simulink model "RoboSoccer"  (R2021b)
settings: Solver=ode15s  StartTime=0.0  StopTime=inf  RelTol=1e-3  EnableMultiTasking=on
PreLoadFcn:
  | load busobjects.mat;
libraries: vrlib x6, simulink x4
settings Model: Creator=smahapat  LastModifiedBy=sarth
settings SolverCC: ZeroCrossControl=DisableAll  AlgebraicLoopSolver=TrustRegion
settings DataIOCC: LimitDataPoints=on  SaveFormat=Array  SignalLoggingSaveFormat=ModelDataLogs  ReturnWorkspaceOutputs=off
settings OptimizationCC: DefaultParameterBehavior=Inlined  ExpressionDepthLimit=2147483647  LifeSpan=inf
settings DebuggingCC: UnderspecifiedInitializationDetection=Classic  MergeDetectMultiDrivingBlocksExec=none  SolverPrmCheckMsg=warning  FcnCallInpInsideContextMsg=warning  StateNameClashWarn=warning  SFUnexpectedBacktrackingDiag=warning  SFNoUnconditionalDefaultTransitionDiag=warning  SFExecutionAtInitializationDiag=none  SFMachineParentedDataDiag=warning  ArithmeticOperatorsInVariantConditions=warning
settings HardwareCC: ProdBitPerPointer=32  ProdBitPerSizeT=32  ProdBitPerPtrDiffT=32  ProdLargestAtomicFloat=None  ProdIntDivRoundTo=Undefined  ProdEndianess=Unspecified  ProdWordSize=32  ProdHWDeviceType=32-bit Generic
settings ModelReferenceCC: PropagateSignalLabelsOutOfModel=off
settings SFSimCC: SimUseLocalCustomCode=off  SimParseCustomCode=off  CustomCodeUndefinedFunction=UseInterfaceOnly
settings RTWCC: RTWUseLocalCustomCode=off
settings CodeAppCC: StateflowObjectComments=on
settings GRTTargetCC: TargetLangStandard=C89/C90 (ANSI)  CombineOutputUpdateFcns=off  GRTInterface=on
settings ConfigComp: CovMetricSettings=dw  CovSaveCumulativeToWorkspaceVar=on  CovSaveSingleToWorkspaceVar=on  CovExternalEMLEnable=off

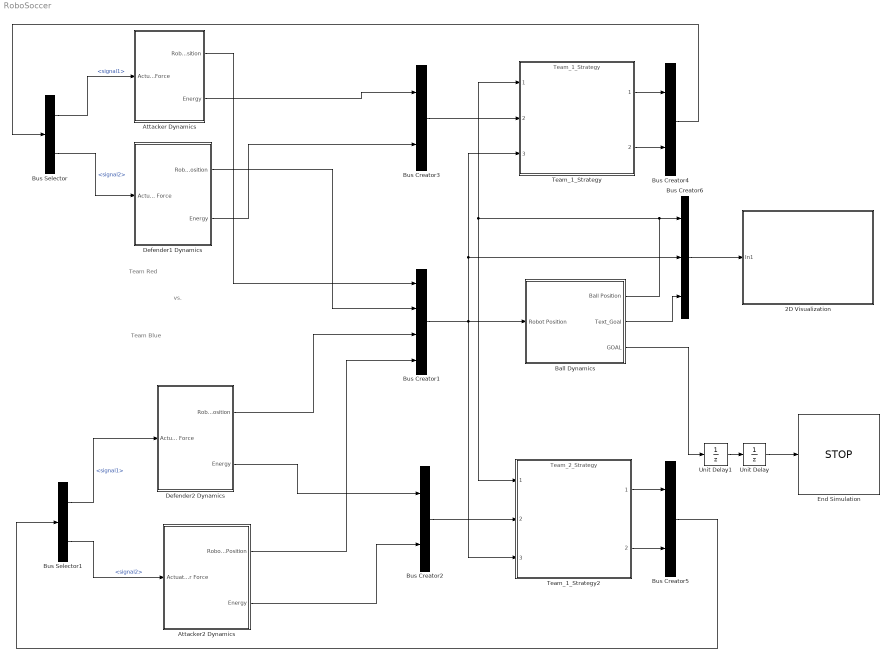
== system RoboSoccer ==
  note: Team Blue
  note: Team Red
  note: vs.
  2D Visualization : Subsystem
      mask Display: image(imread('texture\3D_visualization.jpg'));
  Attacker Dynamics : Subsystem  mask(Robot Parameters){P=0.5, saturate_value=0}
      mask prompts: P "Stamina (Enter value between 0 and 1)"; saturate_value "Actuator_saturation"
      mask help:
      | Set the robot stamina to a value between 0.1 and 1. Note that a higher value of stamina corresponds to more battery power which inversely impacts the mass of the robot. This will reduce its agility.
      |
      | Likewise, higher values of accuracy will come at a cost of higher rates of discharge for the battery pack.
      |
      | Choose values carefully to reflect these tradeoffs.
      mask init:
      | saturate_value=300;
      settings: CloseFcn=|
      | if P<0
      |     error('P cannot be less than 0');
      | end
      | if P>1
      |     error('P cannot be greater than 1');
      | end
      | 
      | if sigma<0
      |     error('sigma cannot be less than 0');
      | end
      | 
      | if sigma>1
      |     error('sigma cannot be greater than 1');
      | end
      mask Help:
      | Set the robot stamina to a value between 0.1 and 1. Note that a higher value of stamina corresponds to more battery power which inversely impacts the mass of the robot. This will reduce its agility.
      | 
      | Likewise, higher values of accuracy will come at a cost of higher rates of discharge for the battery pack.
      | 
      | Choose values carefully to reflect these tradeoffs.
      mask Callback saturate_value: saturate_value=10;
      mask Display: image(imread('texture\Nao6_D.jpeg'));
  Attacker2 Dynamics : Subsystem  mask(Robot Parameters){P=0.5, saturate_value=0}
      mask prompts: P "Stamina (Enter value between 0 and 1)"; saturate_value "Actuator_saturation"
      mask help:
      | Set the robot stamina to a value between 0.1 and 1. Note that a higher value of stamina corresponds to more battery power which inversely impacts the mass of the robot. This will reduce its agility.
      |
      | Likewise, higher values of accuracy will come at a cost of higher rates of discharge for the battery pack.
      |
      | Choose values carefully to reflect these tradeoffs.
      mask init:
      | saturate_value=300;
      settings: CloseFcn=|
      | if P<0
      |     error('P cannot be less than 0');
      | end
      | if P>1
      |     error('P cannot be greater than 1');
      | end
      | 
      | if sigma<0
      |     error('sigma cannot be less than 0');
      | end
      | 
      | if sigma>1
      |     error('sigma cannot be greater than 1');
      | end
      mask Help:
      | Set the robot stamina to a value between 0.1 and 1. Note that a higher value of stamina corresponds to more battery power which inversely impacts the mass of the robot. This will reduce its agility.
      | 
      | Likewise, higher values of accuracy will come at a cost of higher rates of discharge for the battery pack.
      | 
      | Choose values carefully to reflect these tradeoffs.
      mask Callback saturate_value: saturate_value=10;
      mask Display: image(imread('texture\Nao6_D.jpeg'));
  Ball Dynamics : Subsystem  TreatAsAtomicUnit=on
      mask Display: image(imread('texture\soccer_ball_dynamics.jpg'));
  Bus Creator1 : BusCreator  Inputs=4  OutDataTypeStr=Bus: Bus_Robot_Positions
  Bus Creator2 : BusCreator  Inputs=2  OutDataTypeStr=Bus: Bus_Power
  Bus Creator3 : BusCreator  Inputs=2  OutDataTypeStr=Bus: Bus_Power
  Bus Creator4 : BusCreator  Inputs=2
  Bus Creator5 : BusCreator  Inputs=2
  Bus Creator6 : BusCreator  Inputs=3
  Bus Selector : BusSelector  OutputSignals=signal1,signal2
  Bus Selector1 : BusSelector  OutputSignals=signal1,signal2
  Defender1 Dynamics : Subsystem  mask(Robot Parameters){P=0.5, saturate_value=0}
      mask prompts: P "Stamina (Enter value between 0 and 1)"; saturate_value "Actuator_saturation"
      mask help:
      | Set the robot stamina to a value between 0.1 and 1. Note that a higher value of stamina corresponds to more battery power which inversely impacts the mass of the robot. This will reduce its agility.
      |
      | Likewise, higher values of accuracy will come at a cost of higher rates of discharge for the battery pack.
      |
      | Choose values carefully to reflect these tradeoffs.
      mask init:
      | saturate_value=300;
      settings: CloseFcn=|
      | if P<0
      |     error('P cannot be less than 0');
      | end
      | if P>1
      |     error('P cannot be greater than 1');
      | end
      | 
      | if sigma<0
      |     error('sigma cannot be less than 0');
      | end
      | 
      | if sigma>1
      |     error('sigma cannot be greater than 1');
      | end
      mask Help:
      | Set the robot stamina to a value between 0.1 and 1. Note that a higher value of stamina corresponds to more battery power which inversely impacts the mass of the robot. This will reduce its agility.
      | 
      | Likewise, higher values of accuracy will come at a cost of higher rates of discharge for the battery pack.
      | 
      | Choose values carefully to reflect these tradeoffs.
      mask Callback saturate_value: saturate_value=10;
      mask Display: image(imread('texture\Nao6_A.jpeg'));
  Defender2 Dynamics : Subsystem  mask(Robot Parameters){P=0.5, saturate_value=0}
      mask prompts: P "Stamina (Enter value between 0 and 1)"; saturate_value "Actuator_saturation"
      mask help:
      | Set the robot stamina to a value between 0.1 and 1. Note that a higher value of stamina corresponds to more battery power which inversely impacts the mass of the robot. This will reduce its agility.
      |
      | Likewise, higher values of accuracy will come at a cost of higher rates of discharge for the battery pack.
      |
      | Choose values carefully to reflect these tradeoffs.
      mask init:
      | saturate_value=300;
      settings: CloseFcn=|
      | if P<0
      |     error('P cannot be less than 0');
      | end
      | if P>1
      |     error('P cannot be greater than 1');
      | end
      | 
      | if sigma<0
      |     error('sigma cannot be less than 0');
      | end
      | 
      | if sigma>1
      |     error('sigma cannot be greater than 1');
      | end
      mask Help:
      | Set the robot stamina to a value between 0.1 and 1. Note that a higher value of stamina corresponds to more battery power which inversely impacts the mass of the robot. This will reduce its agility.
      | 
      | Likewise, higher values of accuracy will come at a cost of higher rates of discharge for the battery pack.
      | 
      | Choose values carefully to reflect these tradeoffs.
      mask Callback saturate_value: saturate_value=10;
      mask Display: image(imread('texture\Nao6_A.jpeg'));
  End Simulation : Stop
  Team_1_Strategy : ModelReference  ModelNameDialog=Team_1_Strategy  SimulationMode=Normal  ModelReferenceVersion=1.19
      mask Display: image(imread('texture\Strategy.jpg'));
  Team_1_Strategy2 : ModelReference  ModelNameDialog=Team_2_Strategy  SimulationMode=Normal  ModelReferenceVersion=1.24
      mask Display: image(imread('texture\strategy.jpg'));
  Unit Delay : UnitDelay  SampleTime=-1
  Unit Delay1 : UnitDelay  SampleTime=-1
  wires:
  Attacker Dynamics/1(Robot Position) -> Bus Creator1/1
  Defender1 Dynamics/1(Robot Position) -> Bus Creator1/2
  Defender2 Dynamics/1(Robot Position) -> Bus Creator1/3
  Attacker2 Dynamics/1(Robot Position) -> Bus Creator1/4
  Bus Creator1/1 -> Ball Dynamics/1(Robot Position), Bus Creator6/2, Team_1_Strategy/3, Team_1_Strategy2/3
  Defender2 Dynamics/2(Energy) -> Bus Creator2/1
  Attacker2 Dynamics/2(Energy) -> Bus Creator2/2
  Bus Creator2/1 -> Team_1_Strategy2/2
  Team_1_Strategy2/1 -> Bus Creator5/1
  Team_1_Strategy2/2 -> Bus Creator5/2
  Bus Creator5/1 -> Bus Selector1/1
  Team_1_Strategy/1 -> Bus Creator4/1
  Team_1_Strategy/2 -> Bus Creator4/2
  Bus Creator4/1 -> Bus Selector/1
  Bus Selector/1 -> Attacker Dynamics/1(Actuator Force)  "<signal1>"
  Bus Selector/2 -> Defender1 Dynamics/1(Actuator Force)  "<signal2>"
  Bus Selector1/1 -> Defender2 Dynamics/1(Actuator Force)  "<signal1>"
  Bus Selector1/2 -> Attacker2 Dynamics/1(Actuator Force)  "<signal2>"
  Ball Dynamics/3(GOAL) -> Unit Delay1/1
  Ball Dynamics/1(Ball Position) -> Bus Creator6/1, Team_1_Strategy/1, Team_1_Strategy2/1
  Bus Creator6/1 -> 2D Visualization/1(In1)
  Ball Dynamics/2(Text_Goal) -> Bus Creator6/3
  Bus Creator3/1 -> Team_1_Strategy/2
  Defender1 Dynamics/2(Energy) -> Bus Creator3/2
  Attacker Dynamics/2(Energy) -> Bus Creator3/1
  Unit Delay/1 -> End Simulation/1
  Unit Delay1/1 -> Unit Delay/1

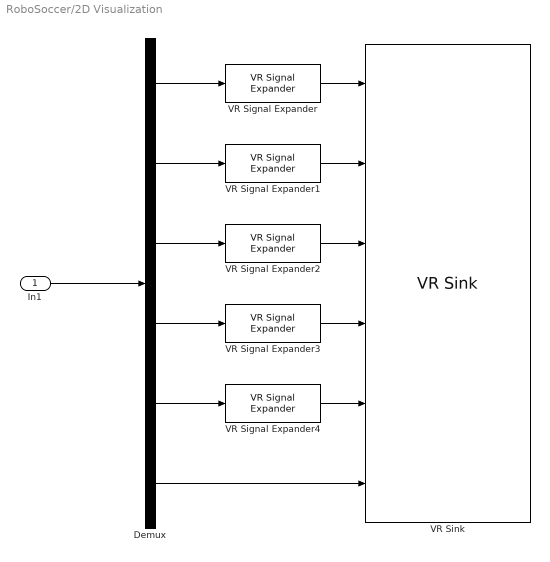
== system RoboSoccer/2D Visualization ==
  In1 : Inport
  Demux : Demux  Outputs=6
  VR Signal Expander{,1..4} (5 alike) : vrlib/VR Signal Expander  outwidth=3  outidx=[1 2]
  VR Sink : vrlib/VR Sink  InstantiateOnLoad=on  SampleTime=0.01  ViewEnable=on  RemoteChange=off  RemoteView=on  FieldsWritten=Ball.translation.3.1.1.double#Robot_1.translation.3.1.1.double#Robot_2.translation.3.1.1.double#Robot_3.translation.3.1.1.double#Robot_4.translation.3.1.1.double#GOAL.translation.3.1.1.double  WorldFileName=robosoccer.WRL  WorldDescription=Robot Soccer Simulator  AutoView=on  VideoDimensions=[]  AllowVariableSize=off
  wires:
  VR Signal Expander/1 -> VR Sink/1
  VR Signal Expander1/1 -> VR Sink/2
  VR Signal Expander2/1 -> VR Sink/3
  VR Signal Expander4/1 -> VR Sink/5
  In1/1 -> Demux/1
  Demux/5 -> VR Signal Expander4/1
  Demux/4 -> VR Signal Expander3/1
  Demux/3 -> VR Signal Expander2/1
  Demux/2 -> VR Signal Expander1/1
  Demux/1 -> VR Signal Expander/1
  VR Signal Expander3/1 -> VR Sink/4
  Demux/6 -> VR Sink/6

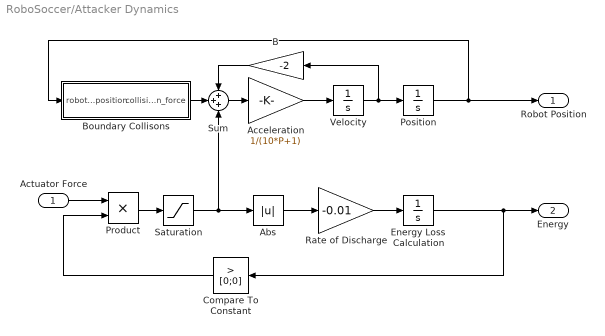
== system RoboSoccer/Attacker Dynamics ==
  Actuator Force : Inport
  Abs : Abs
  Acceleration : Gain  Gain=1/(10*P+1)
  B : Gain  Gain=-2
  Boundary Collisons : MATLAB Function  TreatAsAtomicUnit=on
  Compare To Constant : simulink/Logic and Bit Operations/Compare To Constant  relop=>  const=[0;0]  OutDataTypeStr=uint8
  Energy Loss Calculation : Integrator  InitialCondition=1000*[P; P]
  Position : Integrator  InitialCondition=[50; 75]
  Product : Product  RndMeth=Zero
  Rate of Discharge : Gain  Gain=-0.01
  Saturation : Saturate  UpperLimit=saturate_value  LowerLimit=-saturate_value
  Sum : Sum  Inputs=+++
  Velocity : Integrator  InitialCondition=[0;0]
  Robot Position : Outport  PortDimensions=[2 1]
  Energy : Outport  Port=2  PortDimensions=[2 1]
  wires:
  Acceleration/1 -> Velocity/1
  Velocity/1 -> Position/1, B/1
  Position/1 -> Boundary Collisons/1(robot_position), Robot Position/1
  Energy Loss Calculation/1 -> Energy/1, Compare To Constant/1
  Rate of Discharge/1 -> Energy Loss Calculation/1
  Saturation/1 -> Abs/1, Sum/3
  Abs/1 -> Rate of Discharge/1
  Actuator Force/1 -> Product/1
  Product/1 -> Saturation/1
  Compare To Constant/1 -> Product/2
  Boundary Collisons/1(collision_force) -> Sum/2
  Sum/1 -> Acceleration/1
  B/1 -> Sum/1

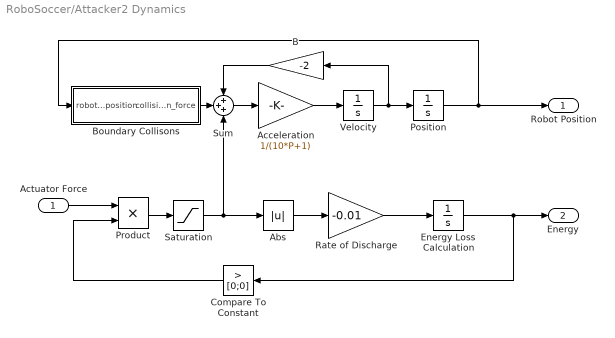
== system RoboSoccer/Attacker2 Dynamics ==
  Actuator Force : Inport
  Abs : Abs
  Acceleration : Gain  Gain=1/(10*P+1)
  B : Gain  Gain=-2
  Boundary Collisons : MATLAB Function  TreatAsAtomicUnit=on
  Compare To Constant : simulink/Logic and Bit Operations/Compare To Constant  relop=>  const=[0;0]  OutDataTypeStr=uint8
  Energy Loss Calculation : Integrator  InitialCondition=1000*[P; P]
  Position : Integrator  InitialCondition=[150; 25]
  Product : Product  RndMeth=Zero
  Rate of Discharge : Gain  Gain=-0.01
  Saturation : Saturate  UpperLimit=saturate_value  LowerLimit=-saturate_value
  Sum : Sum  Inputs=+++
  Velocity : Integrator  InitialCondition=[0;0]
  Robot Position : Outport  PortDimensions=[2 1]
  Energy : Outport  Port=2  PortDimensions=[2 1]
  wires:
  Sum/1 -> Acceleration/1
  Acceleration/1 -> Velocity/1
  Velocity/1 -> Position/1, B/1
  Position/1 -> Boundary Collisons/1(robot_position), Robot Position/1
  Energy Loss Calculation/1 -> Energy/1, Compare To Constant/1
  Rate of Discharge/1 -> Energy Loss Calculation/1
  Saturation/1 -> Abs/1, Sum/3
  Abs/1 -> Rate of Discharge/1
  Actuator Force/1 -> Product/1
  Product/1 -> Saturation/1
  Compare To Constant/1 -> Product/2
  Boundary Collisons/1(collision_force) -> Sum/2
  B/1 -> Sum/1

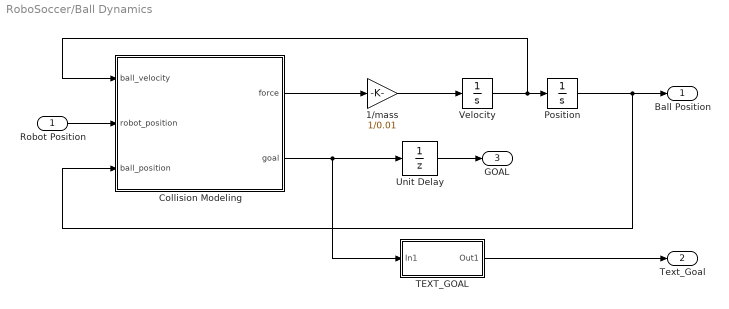
== system RoboSoccer/Ball Dynamics ==
  Robot Position : Inport
  1/mass : Gain  Gain=1/0.01
  Collision Modeling : MATLAB Function  TreatAsAtomicUnit=on
  Position : Integrator  InitialCondition=[100;50]
  TEXT_GOAL : Subsystem
  Unit Delay : UnitDelay  SampleTime=-1
  Velocity : Integrator  InitialCondition=[0;0]
  Ball Position : Outport
  Text_Goal : Outport  Port=2
  GOAL : Outport  Port=3
  wires:
  Robot Position/1 -> Collision Modeling/2(robot_position)
  Velocity/1 -> Position/1, Collision Modeling/1(ball_velocity)
  Position/1 -> Ball Position/1, Collision Modeling/3(ball_position)
  Collision Modeling/1(force) -> 1/mass/1
  1/mass/1 -> Velocity/1
  Collision Modeling/2(goal) -> Unit Delay/1, TEXT_GOAL/1(In1)
  Unit Delay/1 -> GOAL/1
  TEXT_GOAL/1(Out1) -> Text_Goal/1

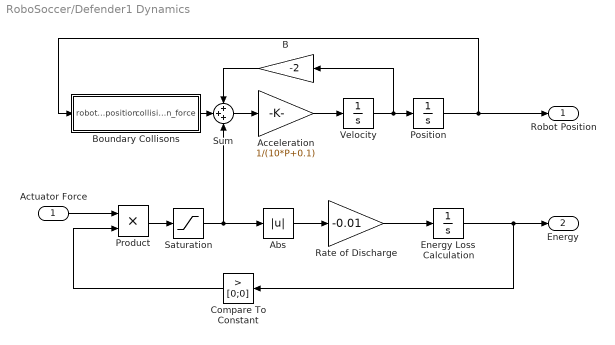
== system RoboSoccer/Defender1 Dynamics ==
  Actuator Force : Inport
  Abs : Abs
  Acceleration : Gain  Gain=1/(10*P+0.1)
  B : Gain  Gain=-2
  Boundary Collisons : MATLAB Function  TreatAsAtomicUnit=on
  Compare To Constant : simulink/Logic and Bit Operations/Compare To Constant  relop=>  const=[0;0]  OutDataTypeStr=uint8
  Energy Loss Calculation : Integrator  InitialCondition=1000*[P; P]
  Position : Integrator  InitialCondition=[50; 25]
  Product : Product  RndMeth=Zero
  Rate of Discharge : Gain  Gain=-0.01
  Saturation : Saturate  UpperLimit=saturate_value  LowerLimit=-saturate_value
  Sum : Sum  Inputs=+++
  Velocity : Integrator  InitialCondition=[0;0]
  Robot Position : Outport  PortDimensions=[2 1]
  Energy : Outport  Port=2  PortDimensions=[2 1]
  wires:
  Compare To Constant/1 -> Product/2
  Product/1 -> Saturation/1
  Actuator Force/1 -> Product/1
  Abs/1 -> Rate of Discharge/1
  Saturation/1 -> Abs/1, Sum/3
  Rate of Discharge/1 -> Energy Loss Calculation/1
  Energy Loss Calculation/1 -> Compare To Constant/1, Energy/1
  Position/1 -> Robot Position/1, Boundary Collisons/1(robot_position)
  Velocity/1 -> Position/1, B/1
  Acceleration/1 -> Velocity/1
  Sum/1 -> Acceleration/1
  Boundary Collisons/1(collision_force) -> Sum/2
  B/1 -> Sum/1

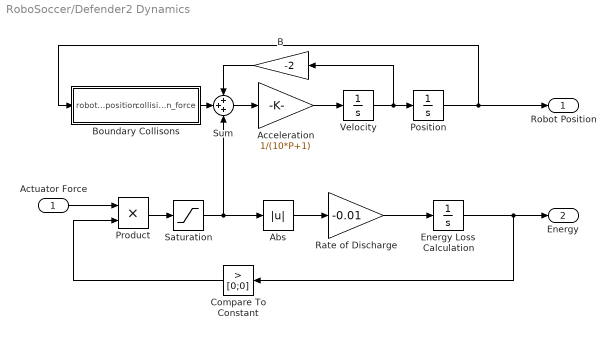
== system RoboSoccer/Defender2 Dynamics ==
  Actuator Force : Inport
  Abs : Abs
  Acceleration : Gain  Gain=1/(10*P+1)
  B : Gain  Gain=-2
  Boundary Collisons : MATLAB Function  TreatAsAtomicUnit=on
  Compare To Constant : simulink/Logic and Bit Operations/Compare To Constant  relop=>  const=[0;0]  OutDataTypeStr=uint8
  Energy Loss Calculation : Integrator  InitialCondition=1000*[P; P]
  Position : Integrator  InitialCondition=[150; 75]
  Product : Product  RndMeth=Zero
  Rate of Discharge : Gain  Gain=-0.01
  Saturation : Saturate  UpperLimit=saturate_value  LowerLimit=-saturate_value
  Sum : Sum  Inputs=+++
  Velocity : Integrator  InitialCondition=[0;0]
  Robot Position : Outport  PortDimensions=[2 1]
  Energy : Outport  Port=2  PortDimensions=[2 1]
  wires:
  Compare To Constant/1 -> Product/2
  Product/1 -> Saturation/1
  Actuator Force/1 -> Product/1
  Abs/1 -> Rate of Discharge/1
  Saturation/1 -> Abs/1, Sum/3
  Rate of Discharge/1 -> Energy Loss Calculation/1
  Energy Loss Calculation/1 -> Compare To Constant/1, Energy/1
  Position/1 -> Robot Position/1, Boundary Collisons/1(robot_position)
  Velocity/1 -> Position/1, B/1
  Acceleration/1 -> Velocity/1
  Sum/1 -> Acceleration/1
  Boundary Collisons/1(collision_force) -> Sum/2
  B/1 -> Sum/1

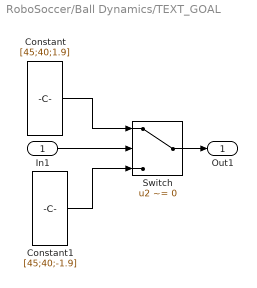
== system RoboSoccer/Ball Dynamics/TEXT_GOAL ==
  In1 : Inport
  Constant : Constant  Value=[45;40;1.9]
  Constant1 : Constant  Value=[45;40;-1.9]
  Switch : Switch  Criteria=u2 ~= 0  Threshold=1
  Out1 : Outport
  wires:
  In1/1 -> Switch/2
  Switch/1 -> Out1/1
  Constant/1 -> Switch/1
  Constant1/1 -> Switch/3

== matlab function RoboSoccer/Ball Dynamics/Collision Modeling ==
  data: ball_velocity input; robot_position input size=[8 ;1]; ball_position input size=[2;1]; force output size=[2;1]; goal output
function [force, goal] = fcn(ball_velocity,robot_position, ball_position)
%#eml
% Initialize variables

force1=zeros(2,1);
force2=zeros(2,1);
force3=zeros(2,1);
force4=zeros(2,1);
collision_force=zeros(2,1);
d1=zeros(2,1);
d2=zeros(2,1);
d3=zeros(2,1);
d4=zeros(2,1);
K=100;
goal=0;
tol=25;
B=0.01;

% Compute dot products and calculate impulsive forces on the ball
d1=robot_position(1:2,1)-ball_position;
d2=robot_position(3:4,1)-ball_position;
d3=robot_position(5:6,1)-ball_position;
d4=robot_position(7:8,1)-ball_position;

if   dot(d1,d1) <tol
     force1=-K*d1;
end

if   dot(d2,d2) <tol
     force2=-K*d2;
end

if   dot(d3,d3) <tol
     force3=-K*d3;
end

if   dot(d4,d4) <tol
     force4=-K*d4;
end

% Code to check for boundary collisions for the ball
if ball_position(1,1)<0 
    collision_force(1,1)=-K*ball_position(1,1);
end

if ball_position(1,1)>200 
    collision_force(1,1)=K*(200-ball_position(1,1));
end

if ball_position(2,1)<0 
    collision_force(2,1)=-K*ball_position(2,1);
end

if ball_position(2,1)>100 
    collision_force(2,1)=K*(100-ball_position(2,1)); 
end

% Total force
force=collision_force+force1+force2+force3+force4-B*ball_velocity;

% Goal scored
if ((ball_position(1,1)<=0) && (ball_position(2,1)>41) && (ball_position(2,1)<59))
    goal=1; 
end

if ((ball_position(1,1)>=200) && (ball_position(2,1)>41) && (ball_position(2,1)<59))
    goal=1; 
end

== matlab function RoboSoccer/Attacker Dynamics/Boundary Collisons ==
  data: robot_position input; collision_force output
function collision_force = fcn(robot_position)
%#eml
K=100;
collision_force=[0; 0]; 
if robot_position(1,1)<0 
    collision_force(1,1)=-K*robot_position(1,1);
end

if robot_position(1,1)>200 
    collision_force(1,1)=K*(200-robot_position(1,1));
end

if robot_position(2,1)<0 
    collision_force(2,1)=-K*robot_position(2,1);
end

if robot_position(2,1)>100 
    collision_force(2,1)=K*(100-robot_position(2,1));
end

== matlab function RoboSoccer/Attacker2 Dynamics/Boundary Collisons ==
  data: robot_position input; collision_force output
function collision_force = fcn(robot_position)
%#eml
K=100;
collision_force=[0; 0]; 
if robot_position(1,1)<0 
    collision_force(1,1)=-K*robot_position(1,1);
end

if robot_position(1,1)>200 
    collision_force(1,1)=K*(200-robot_position(1,1));
end

if robot_position(2,1)<0 
    collision_force(2,1)=-K*robot_position(2,1);
end

if robot_position(2,1)>100 
    collision_force(2,1)=K*(100-robot_position(2,1));
end

== matlab function RoboSoccer/Defender2 Dynamics/Boundary Collisons ==
  data: robot_position input; collision_force output
function collision_force = fcn(robot_position)
%#eml
K=100;
collision_force=[0; 0]; 
if robot_position(1,1)<0 
    collision_force(1,1)=-K*robot_position(1,1);
end

if robot_position(1,1)>200 
    collision_force(1,1)=K*(200-robot_position(1,1));
end

if robot_position(2,1)<0 
    collision_force(2,1)=-K*robot_position(2,1);
end

if robot_position(2,1)>100 
    collision_force(2,1)=K*(100-robot_position(2,1));
end

== matlab function RoboSoccer/Defender1 Dynamics/Boundary Collisons ==
  data: robot_position input; collision_force output
function collision_force = fcn(robot_position)
%#eml
K=100;
collision_force=[0; 0]; 
if robot_position(1,1)<0 
    collision_force(1,1)=-K*robot_position(1,1);
end

if robot_position(1,1)>200 
    collision_force(1,1)=K*(200-robot_position(1,1));
end

if robot_position(2,1)<0 
    collision_force(2,1)=-K*robot_position(2,1);
end

if robot_position(2,1)>100 
    collision_force(2,1)=K*(100-robot_position(2,1));
end
